simulink model "IT1_FPID_Controller"  (R2024a)
settings: Solver=ode4  StartTime=0.0  StopTime=8  FixedStep=0.05  RelTol=1e-3  EnableMultiTasking=on
values from neighbouring files (symbols this model uses):
  K = 1    [runControlSystemExample_FIS1.m]
  Ka = 0.077    [runControlSystemExample_FIS1.m]
  Kb = 7.336    [runControlSystemExample_FIS1.m]
  Kd = 0.5141    [runControlSystemExample_FIS1.m]
  Ke = 1    [runControlSystemExample_FIS1.m]
  L = 0.3    [runControlSystemExample_FIS1.m]
  T = 1.1    [runControlSystemExample_FIS1.m]
libraries: fuzblock x1
settings Model: Creator=u11f99  LastModifiedBy=ilicm
settings SolverCC: AlgebraicLoopSolver=TrustRegion
settings DataIOCC: LimitDataPoints=on  SaveFormat=Array  ReturnWorkspaceOutputs=off
settings OptimizationCC: ExpressionDepthLimit=2147483647  LifeSpan=inf
settings DebuggingCC: UnderspecifiedInitializationDetection=Classic  MergeDetectMultiDrivingBlocksExec=none  SolverPrmCheckMsg=warning  UnconnectedInputMsg=warning  UnconnectedOutputMsg=warning  UnconnectedLineMsg=warning  AllowSymbolicDim=off  StateNameClashWarn=warning  SFUnexpectedBacktrackingDiag=warning  SFNoUnconditionalDefaultTransitionDiag=warning  SFExecutionAtInitializationDiag=none  ArithmeticOperatorsInVariantConditions=warning
settings HardwareCC: ProdBitPerPointer=32  ProdBitPerSizeT=32  ProdBitPerPtrDiffT=32  ProdLargestAtomicFloat=None  ProdIntDivRoundTo=Undefined  ProdEndianess=Unspecified  ProdWordSize=32  ProdHWDeviceType=32-bit Generic
settings ModelReferenceCC: EnableRefExpFcnMdlSchedulingChecks=on  PropagateSignalLabelsOutOfModel=off
settings SFSimCC: SimUseLocalCustomCode=off  CustomCodeUndefinedFunction=UseInterfaceOnly
settings RTWCC: RTWUseLocalCustomCode=off  GPUComputeCapability=3.5
settings CodeAppCC: StateflowObjectComments=on
settings GRTTargetCC: TargetLangStandard=C89/C90 (ANSI)
settings ConfigComp: CovMetricSettings=dw  CovSaveCumulativeToWorkspaceVar=on  CovSaveSingleToWorkspaceVar=on  CovExternalEMLEnable=off

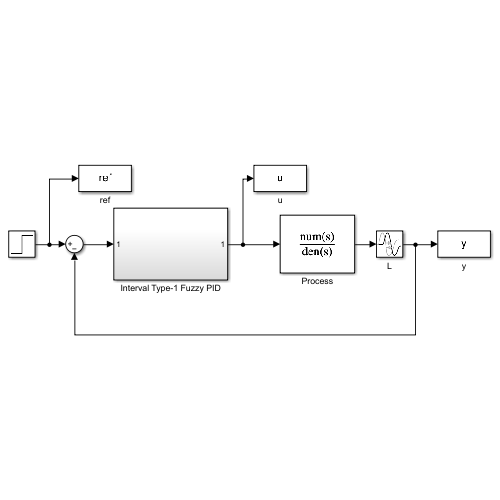
[thumbnail: Simulink's stored preview of the top-level diagram]
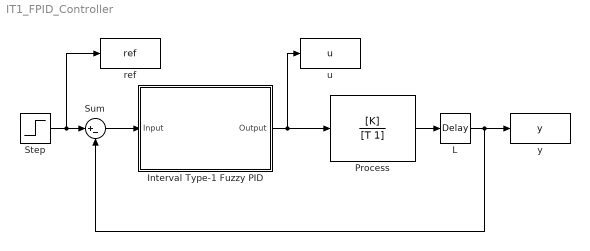
== system IT1_FPID_Controller ==
  Interval Type-1 Fuzzy PID : Subsystem
  L : TransportDelay  DelayTime=L
  Process : TransferFcn  Numerator=[K]  Denominator=[T 1]
  Step : Step  SampleTime=0
  Sum : Sum  Inputs=|+-
  ref : ToWorkspace  VariableName=ref  SaveFormat=Structure With Time  SampleTime=-1
  u : ToWorkspace  VariableName=u  SaveFormat=Structure With Time  SampleTime=-1
  y : ToWorkspace  VariableName=y  SaveFormat=Structure With Time  SampleTime=-1
  wires:
  Step/1 -> ref/1, Sum/1
  Sum/1 -> Interval Type-1 Fuzzy PID/1(Input)
  Process/1 -> L/1
  L/1 -> Sum/2, y/1
  Interval Type-1 Fuzzy PID/1(Output) -> u/1, Process/1

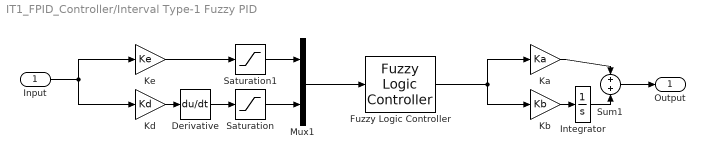
== system IT1_FPID_Controller/Interval Type-1 Fuzzy PID ==
  Input : Inport
  Derivative : Derivative
  Fuzzy Logic Controller : fuzblock/Fuzzy Logic  Controller  FIS='FIS_t1.fis'  OutputSampleNumber=101  DataType=double  FuzzifiedInputs=off  RuleFiringStrengths=off  RuleOutputs=off  AggregatedOutputs=off  SimulateUsing=Interpreted execution  OutOfRangeInputValueMessage=warning  NoRuleFiredMessage=warning  EmptyOutputFuzzySetMessage=warning
  Integrator : Integrator
  Ka : Gain  Gain=Ka
  Kb : Gain  Gain=Kb
  Kd : Gain  Gain=Kd
  Ke : Gain  Gain=Ke
  Mux1 : Mux  Inputs=2
  Saturation : Saturate  UpperLimit=1  LowerLimit=-1
  Saturation1 : Saturate  UpperLimit=1  LowerLimit=-1
  Sum1 : Sum
  Output : Outport
  wires:
  Saturation1/1 -> Mux1/1
  Saturation/1 -> Mux1/2
  Derivative/1 -> Saturation/1
  Kd/1 -> Derivative/1
  Ke/1 -> Saturation1/1
  Input/1 -> Kd/1, Ke/1
  Fuzzy Logic Controller/1 -> Kb/1, Ka/1
  Kb/1 -> Integrator/1
  Integrator/1 -> Sum1/2
  Ka/1 -> Sum1/1
  Sum1/1 -> Output/1
  Mux1/1 -> Fuzzy Logic Controller/1
